simulink model "lab2s2022a"  (R2022a)
settings: Solver=VariableStepAuto  StartTime=0.0  StopTime=Tmdl  RelTol=1e-3
undefined symbols (not defined in the file): J, k, Lex, r1, r2, r3, Ra, radd, Rex, Tload, ua, Ua_change, ue
libraries: fl_lib x17, nesl_utility x12
settings Model: Creator=86156  LastModifiedBy=86156
settings DebuggingCC: AlgebraicLoopMsg=none
settings ModelReferenceCC: EnableRefExpFcnMdlSchedulingChecks=off
settings RTWCC: Description=Generic Real-Time Target

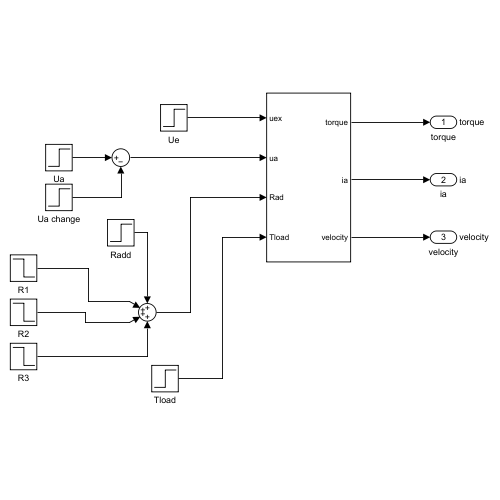
[thumbnail: Simulink's stored preview of the top-level diagram]
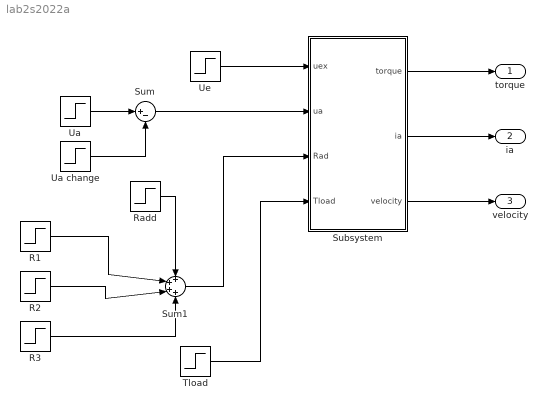
== system lab2s2022a ==
  R1 : Step  Time=10  Before=r1  After=0  SampleTime=0
  R2 : Step  Time=25  Before=r2  After=0  SampleTime=0
  R3 : Step  Time=40  Before=r3  After=0  SampleTime=0
  Radd : Step  Time=50  After=radd  SampleTime=0
  Subsystem : Subsystem
  Sum : Sum  Inputs=|+-
  Sum1 : Sum  Inputs=++++
  Tload : Step  After=Tload  SampleTime=0
  Ua : Step  After=ua  SampleTime=0
  Ua change : Step  Time=50  After=Ua_change  SampleTime=0
  Ue : Step  Time=0  After=ue  SampleTime=0
  torque : Outport  SignalName=torque
  ia : Outport  Port=2  SignalName=ia
  velocity : Outport  Port=3  SignalName=velocity
  wires:
  Ue/1 -> Subsystem/1(uex)
  Subsystem/1(torque) -> torque/1
  Subsystem/2(ia) -> ia/1
  Subsystem/3(velocity) -> velocity/1
  Tload/1 -> Subsystem/4(Tload)
  Ua change/1 -> Sum/2
  Ua/1 -> Sum/1
  Sum/1 -> Subsystem/2(ua)
  R1/1 -> Sum1/2
  Radd/1 -> Sum1/1
  R2/1 -> Sum1/3
  R3/1 -> Sum1/4
  Sum1/1 -> Subsystem/3(Rad)

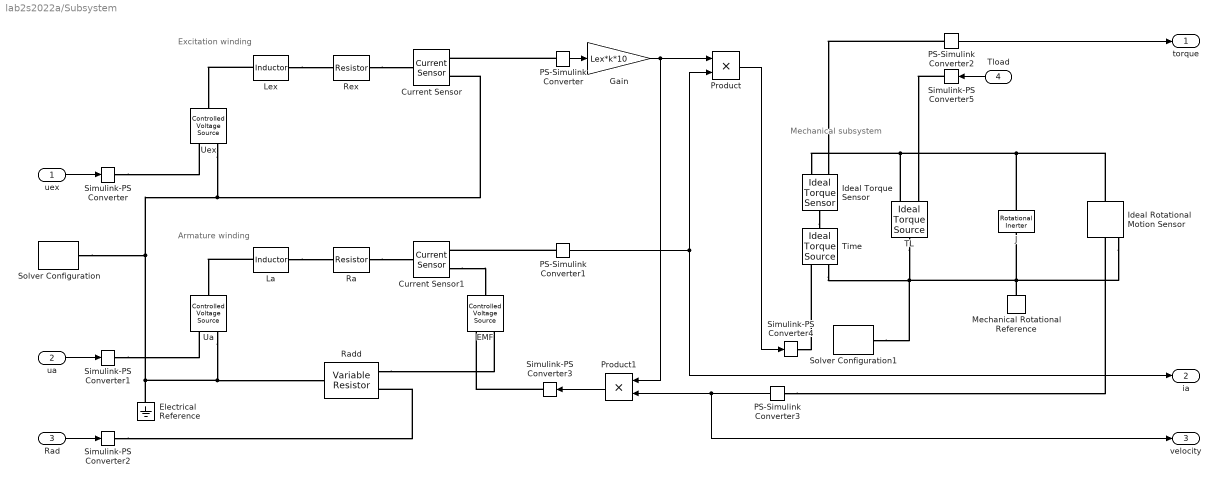
== system lab2s2022a/Subsystem ==
  note: Excitation winding
  note: Armature winding
  note: Mechanical subsystem
  uex : Inport
  ua : Inport  Port=2
  Rad : Inport  Port=3
  Tload : Inport  Port=4
  " Time" : fl_lib/Mechanical/Mechanical Sources/Ideal Torque Source
  Current Sensor : fl_lib/Electrical/Electrical Sensors/Current Sensor
  Current Sensor1 : fl_lib/Electrical/Electrical Sensors/Current Sensor
  EMF : fl_lib/Electrical/Electrical Sources/Controlled Voltage Source
  Electrical Reference : fl_lib/Electrical/Electrical Elements/Electrical Reference
  Gain : Gain  Gain=Lex*k*10
  Ideal Rotational Motion Sensor : fl_lib/Mechanical/Mechanical Sensors/Ideal Rotational Motion Sensor  reference=foundation.enum.MeasurementReference.difference  acceleration_port=false  velocity_port=true  position_port=true  wrap_angle=simscape.enum.onoff.off  offset=0 rad
  Ideal Torque Sensor : fl_lib/Mechanical/Mechanical Sensors/Ideal Torque Sensor
  J : fl_lib/Mechanical/Rotational Elements/Rotational Inerter  B=J kg*m^2  w_specify=off  w_priority=High  w=0 rad/s  w_nominal_specify=off  w_nominal_unit=rad/s  w_nominal_value=1  t_specify=off  t_priority=None  t=0 N*m  t_nominal_specify=off  t_nominal_unit=N*m  t_nominal_value=1
      settings: InternalSimscapePortConfiguration="{\"Bottom\":[],\"Left\":[{\"id\":\"R\",\"label\":\"R\",\"type\":\"foundation.mechanical.rotational.rotational\"}],\"Right\":[{\"id\":\"C\",\"label\":\"C\",\"type\":\"foundation.mechanical.rotational.rotational\"}],\"Top\":[]}"
  La : fl_lib/Electrical/Electrical Elements/Inductor  l=La H  r=0 Ohm  g=1e-9 1/Ohm  i_specify=off  i_priority=None  i=0 A  i_nominal_specify=off  i_nominal_unit=A  i_nominal_value=1  v_specify=off  v_priority=None  v=0 V  v_nominal_specify=off  v_nominal_unit=V  v_nominal_value=1  i_L_specify=off  i_L_priority=High  i_L=0 A  i_L_nominal_specify=off  i_L_nominal_unit=A  i_L_nominal_value=1
  Lex : fl_lib/Electrical/Electrical Elements/Inductor  l=Lex H  r=0 Ohm  g=1e-9 1/Ohm  i_specify=off  i_priority=None  i=0 A  i_nominal_specify=off  i_nominal_unit=A  i_nominal_value=1  v_specify=off  v_priority=None  v=0 V  v_nominal_specify=off  v_nominal_unit=V  v_nominal_value=1  i_L_specify=off  i_L_priority=High  i_L=0 A  i_L_nominal_specify=off  i_L_nominal_unit=A  i_L_nominal_value=1
  Mechanical Rotational Reference : fl_lib/Mechanical/Rotational Elements/Mechanical Rotational Reference
  PS-Simulink Converter{,1..3} (4 alike) : nesl_utility/PS-Simulink Converter  PhysicalDomain=network_engine_domain  SubClassName=ps_output  LeftPortType=input  RightPortType=output  PseudoPeriodic=off  Frequencies=[]  VectorFormat=1-D array  Unit=inherit  AffineConversion=off
  Product : Product
  Product1 : Product
  Ra : fl_lib/Electrical/Electrical Elements/Resistor  R=Ra Ohm  i_specify=off  i_priority=None  i=0 A  i_nominal_specify=off  i_nominal_unit=A  i_nominal_value=1  v_specify=off  v_priority=None  v=0 V  v_nominal_specify=off  v_nominal_unit=V  v_nominal_value=1
  Radd : fl_lib/Electrical/Electrical Elements/Variable Resistor  Rmin=0 Ohm  i_specify=off  i_priority=None  i=0 A  i_nominal_specify=off  i_nominal_unit=A  i_nominal_value=1  v_specify=off  v_priority=None  v=0 V  v_nominal_specify=off  v_nominal_unit=V  v_nominal_value=1
  Rex : fl_lib/Electrical/Electrical Elements/Resistor  R=Rex Ohm  i_specify=off  i_priority=None  i=0 A  i_nominal_specify=off  i_nominal_unit=A  i_nominal_value=1  v_specify=off  v_priority=None  v=0 V  v_nominal_specify=off  v_nominal_unit=V  v_nominal_value=1
  Simulink-PS Converter{,1..5} (6 alike) : nesl_utility/Simulink-PS Converter  PhysicalDomain=network_engine_domain  SubClassName=ps_input  LeftPortType=input  RightPortType=output  PseudoPeriodic=off  Frequencies=[]  NoiseDistribution=none  NoiseParameters=[]  Unit=1  AffineConversion=off  FilteringAndDerivatives=provide  SimscapeFilterOrder=1  InputFilterTimeConstant=0.001  UdotUserProvided=0
  Solver Configuration : nesl_utility/Solver Configuration  PhysicalDomain=network_engine_domain  SubClassName=solver  LeftPortType=input  RightPortType=generic  Tones=[]  Harmonics=[]  SimulateNoise=off  Profile=off  UseLocalSampling=off  EnableSwitchedLinearOptims=on  FrequencyDomain=off  UseCCode=off  RelTol=0.001  AbsTol=1e-06  MinStep=1e-09  ToWorkspace=off  RevertToSquareIcSolve=off  NumHomotopyIterations=100  PhasorMode=off  PhasorModeNumHarmonics=1  ConsistencySolver=NEWTON_FTOL  IndexReductionMethod=DerivativeReplacement  DoDC=off  ResidualTolerance=1e-09  ConsistencyTolSource=GLOBAL  ConsistencyAbsTol=0.001  ConsistencyRelTol=0.001  ConsistencyTolFactor=0.001  UseLocalSolver=off  LocalSolverChoice=NE_BACKWARD_EULER_ADVANCER  ResolveIndetEquations=on  FunctionEvalNumThread=1  LocalSolverSampleTime=0.001  DoFixedCost=off  MaxNonlinIter=3  MaxModeIter=2  ComputeImpulses=off  ImpulseIterations=2  LinearAlgebra=auto  LinearAlgebraNumThread=0  EquationFormulation=NE_TIME_EF  DelaysMemoryBudget=1024  AutomaticFiltering=on  FilteringTimeConstant=0.001  PartitionStorageMethod=AS_NEEDED  PartitionMemoryBudget=1024  PartitionMethod=ROBUST
  Solver Configuration1 : nesl_utility/Solver Configuration  PhysicalDomain=network_engine_domain  SubClassName=solver  LeftPortType=input  RightPortType=generic  Tones=[]  Harmonics=[]  SimulateNoise=off  Profile=off  UseLocalSampling=off  EnableSwitchedLinearOptims=on  FrequencyDomain=off  UseCCode=off  RelTol=0.001  AbsTol=1e-06  MinStep=1e-09  ToWorkspace=off  RevertToSquareIcSolve=off  NumHomotopyIterations=100  PhasorMode=off  PhasorModeNumHarmonics=1  ConsistencySolver=NEWTON_FTOL  IndexReductionMethod=DerivativeReplacement  DoDC=off  ResidualTolerance=1e-09  ConsistencyTolSource=GLOBAL  ConsistencyAbsTol=0.001  ConsistencyRelTol=0.001  ConsistencyTolFactor=0.001  UseLocalSolver=off  LocalSolverChoice=NE_BACKWARD_EULER_ADVANCER  ResolveIndetEquations=on  FunctionEvalNumThread=1  LocalSolverSampleTime=0.001  DoFixedCost=off  MaxNonlinIter=3  MaxModeIter=2  ComputeImpulses=off  ImpulseIterations=2  LinearAlgebra=auto  LinearAlgebraNumThread=0  EquationFormulation=NE_TIME_EF  DelaysMemoryBudget=1024  AutomaticFiltering=on  FilteringTimeConstant=0.001  PartitionStorageMethod=AS_NEEDED  PartitionMemoryBudget=1024  PartitionMethod=ROBUST
  TL : fl_lib/Mechanical/Mechanical Sources/Ideal Torque Source
  Ua : fl_lib/Electrical/Electrical Sources/Controlled Voltage Source
  Uex : fl_lib/Electrical/Electrical Sources/Controlled Voltage Source
  torque : Outport
  ia : Outport  Port=2
  velocity : Outport  Port=3
  wires:
  Product1/1 -> Simulink-PS Converter3/1
  Tload/1 -> Simulink-PS Converter5/1
  PS-Simulink Converter1/1 -> ia/1, Product/2
  Gain/1 -> Product1/1, Product/1
  Rad/1 -> Simulink-PS Converter2/1
  ua/1 -> Simulink-PS Converter1/1
  PS-Simulink Converter2/1 -> torque/1
  PS-Simulink Converter/1 -> Gain/1
  PS-Simulink Converter3/1 -> velocity/1, Product1/2
  Product/1 -> Simulink-PS Converter4/1
  uex/1 -> Simulink-PS Converter/1
  connections:
  PS-Simulink Converter/LConn1 -- Current Sensor/RConn1
  Ideal Torque Sensor/LConn1 -- " Time"/LConn1
  Ua/RConn2 -- Radd/RConn1 -- Electrical Reference/LConn1 -- Uex/RConn2 -- Current Sensor/RConn2 -- Solver Configuration/RConn1
  Current Sensor1/RConn2 -- EMF/LConn1
  Ra/RConn1 -- Current Sensor1/LConn1
  Ideal Rotational Motion Sensor/RConn1 -- Mechanical Rotational Reference/LConn1 -- J/RConn1 -- Solver Configuration1/RConn1 -- TL/LConn1 -- " Time"/RConn2
  Simulink-PS Converter5/RConn1 -- TL/RConn1
  La/RConn1 -- Ra/LConn1
  J/LConn1 -- Ideal Rotational Motion Sensor/LConn1 -- TL/RConn2 -- Ideal Torque Sensor/RConn1
  Simulink-PS Converter/RConn1 -- Uex/RConn1
  Simulink-PS Converter2/RConn1 -- Radd/LConn1
  Simulink-PS Converter4/RConn1 -- " Time"/RConn1
  Lex/LConn1 -- Uex/LConn1
  Rex/RConn1 -- Current Sensor/LConn1
  PS-Simulink Converter3/LConn1 -- Ideal Rotational Motion Sensor/RConn2
  PS-Simulink Converter1/LConn1 -- Current Sensor1/RConn1
  Radd/LConn2 -- EMF/RConn2
  PS-Simulink Converter2/LConn1 -- Ideal Torque Sensor/RConn2
  Simulink-PS Converter3/RConn1 -- EMF/RConn1
  Simulink-PS Converter1/RConn1 -- Ua/RConn1
  Lex/RConn1 -- Rex/LConn1
  La/LConn1 -- Ua/LConn1
